simulink model "lab12_AM_modulation"  (R2015a)
settings: Solver=ode45  StartTime=0.0  StopTime=10.0  RelTol=1e-3
settings Model: Creator=Hp  LastModifiedBy=Hp

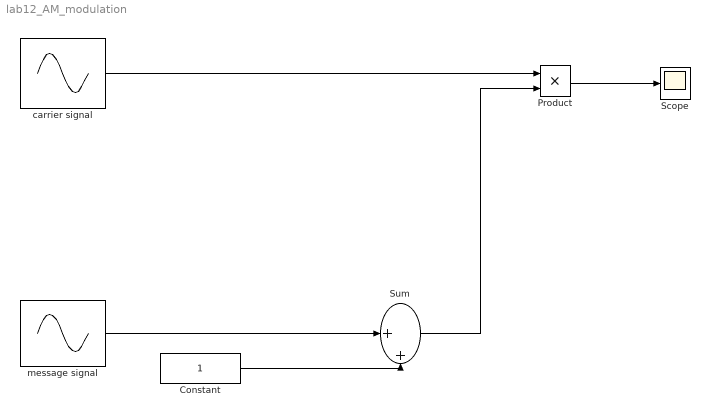
== system lab12_AM_modulation ==
  Constant : Constant
  Product : Product
  Scope : Scope
  Sum : Sum  Inputs=|++
  carrier signal : Sin  Frequency=1000  SampleTime=0.001
  "message signal " : Sin  Amplitude=0.5  Frequency=10  SampleTime=0.01
  wires:
  "message signal "/1 -> Sum/1
  Constant/1 -> Sum/2
  carrier signal/1 -> Product/1
  Sum/1 -> Product/2
  Product/1 -> Scope/1
